simulink model "Plant_development"  (R2022b)
settings: Solver=VariableStepAuto  StartTime=0.0  StopTime=10  RelTol=1e-3
libraries: instrumentlib x2
settings Model: Creator=ariar  LastModifiedBy=NICOLAS
settings DebuggingCC: UnconnectedInputMsg=warning  UnconnectedOutputMsg=warning  UnconnectedLineMsg=warning
settings ModelReferenceCC: EnableRefExpFcnMdlSchedulingChecks=on
settings RTWCC: DLArmComputeVersion=19.05

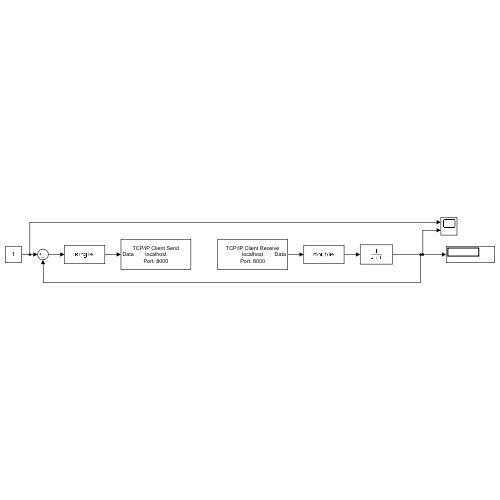
[thumbnail: Simulink's stored preview of the top-level diagram]
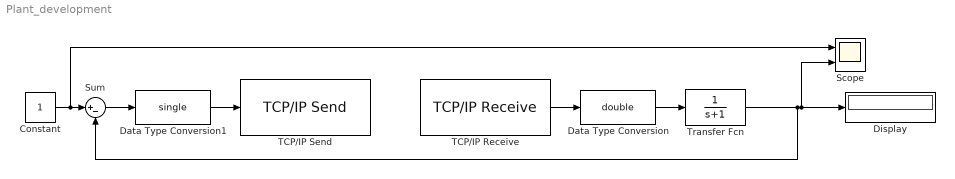
== system Plant_development ==
  Constant : Constant
  Data Type Conversion : DataTypeConversion  OutDataTypeStr=double  SaturateOnIntegerOverflow=off  RndMeth=Floor
  Data Type Conversion1 : DataTypeConversion  OutDataTypeStr=single  SaturateOnIntegerOverflow=off  RndMeth=Floor
  Display : Display
  Scope : Scope  NumInputPorts=2
  Sum : Sum  Inputs=|+-
  TCP/IP Receive : instrumentlib/TCP//IP Receive  Host=localhost  Port=8000  DataSize=[ 1, 1 ]  DataType=single  ASCIIFormatting=%f  Terminator=LF  CustomTerminator=10  ByteOrder=big-endian  EnableBlockingMode=on  Timeout=10  SampleTime=0.01  SimulateUsing=Interpreted execution
  TCP/IP Send : instrumentlib/TCP//IP Send  Host=localhost  Port=8000  ByteOrder=big-endian  EnableBlockingMode=on  Timeout=10  TransferDelay=on  SimulateUsing=Interpreted execution
  Transfer Fcn : TransferFcn  Denominator=[1 1]
  wires:
  TCP/IP Receive/1 -> Data Type Conversion/1
  Data Type Conversion/1 -> Transfer Fcn/1
  Data Type Conversion1/1 -> TCP/IP Send/1
  Transfer Fcn/1 -> Sum/2, Scope/2, Display/1
  Constant/1 -> Scope/1, Sum/1
  Sum/1 -> Data Type Conversion1/1
